simulink model "RebeccaGroup (1)"  (R2020b)
settings: Solver=VariableStepAuto  StartTime=0.0  StopTime=100  RelTol=1e-3
undefined symbols (not defined in the file): LQR
libraries: pid_lib x1
settings Model: Creator=user  LastModifiedBy=user

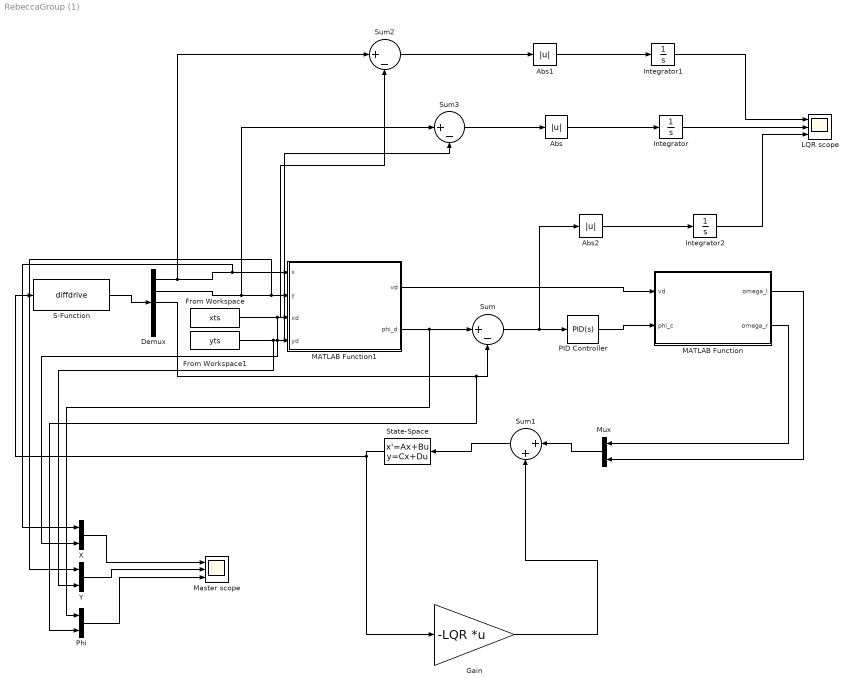
== system RebeccaGroup (1) ==
  Abs : Abs
  Abs1 : Abs
  Abs2 : Abs
  Demux : Demux  Outputs=5
  From Workspace : FromWorkspace  VariableName=xts
  From Workspace1 : FromWorkspace  VariableName=yts
  Gain : Gain  Gain=-LQR  Multiplication=Matrix(K*u)
  Integrator : Integrator
  Integrator1 : Integrator
  Integrator2 : Integrator
  LQR scope : Scope  NumInputPorts=3
  MATLAB Function : MATLAB Function  TreatAsAtomicUnit=on
  MATLAB Function1 : MATLAB Function  TreatAsAtomicUnit=on
  Master scope : Scope  NumInputPorts=3
  Mux : Mux  Inputs=2
  PID Controller : pid_lib/PID Controller  Controller=PID  Form=Parallel  TimeDomain=Continuous-time  UseExternalTs=off  SampleTime=-1  IntegratorMethod=Forward Euler  FilterMethod=Forward Euler  ControllerParametersSource=internal  P=7.98978366638355  I=11.7417923177331  D=0.804824840829485  UseFilter=on  N=170.651260101188  TunerSelectOption=Transfer Function Based (PID Tuner App)  InitialConditionSource=internal  InitialConditionForIntegrator=0  InitialConditionForFilter=0  DifferentiatorICPrevScaledInput=0  ExternalReset=none  TrackingMode=off  Kt=1  LimitOutput=off  SatLimitsSource=internal  UpperSaturationLimit=inf  LowerSaturationLimit=-inf  LinearizeAsGain=on  AntiWindupMode=none  Kb=1  POutMin=[]  POutMax=[]  IOutMin=[]  IOutMax=[]  DOutMin=[]  DOutMax=[]  NOutMin=[]  NOutMax=[]  SumOutMin=[]  SumOutMax=[]  SaturationOutMin=[]  SaturationOutMax=[]  PParamMin=[]  PParamMax=[]  IParamMin=[]  IParamMax=[]  DParamMin=[]  DParamMax=[]  NParamMin=[]  NParamMax=[]  KbParamMin=[]  KbParamMax=[]  KtParamMin=[]  KtParamMax=[]  KbOutMin=[]  KbOutMax=[]  KtOutMin=[]  KtOutMax=[]  IntegratorOutMin=[]  IntegratorOutMax=[]  FilterOutMin=[]  FilterOutMax=[]  SumI1OutMin=[]  SumI1OutMax=[]  SumI2OutMin=[]  SumI2OutMax=[]  SumI3OutMin=[]  SumI3OutMax=[]  SumI4OutMin=[]  SumI4OutMax=[]  SumDOutMin=[]  SumDOutMax=[]  DifferentiatorOutMin=[]  DifferentiatorOutMax=[]  FilterDiffOutCoefMin=[]  FilterDiffOutCoefMax=[]  ReciprocalOutMin=[]  ReciprocalOutMax=[]  SumDenOutMin=[]  SumDenOutMax=[]  SumNumOutMin=[]  SumNumOutMax=[]  DivideOutMin=[]  DivideOutMax=[]  UdiffTsProdOutMin=[]  UdiffTsProdOutMax=[]  NTsProdOutMin=[]  NTsProdOutMax=[]  UintegralTsProdOutMin=[]  UintegralTsProdOutMax=[]  UngainTsProdOutMin=[]  UngainTsProdOutMax=[]  IntegratorContinuousStateAttributes=''  IntegratorStateMustResolveToSignalObject=off  IntegratorRTWStateStorageClass=Auto  FilterContinuousStateAttributes=''  FilterStateMustResolveToSignalObject=off  FilterRTWStateStorageClass=Auto  ParallelPVariant=InternalParameters  IdealPVariant=Disabled  IVariant=InternalParameters  DVariant=InternalParameters  IntegratorVariant=Continuous  SatVariant=Disabled  AWVariant=Passthrough  PCopyVariant=Disabled  TRVariant=Disabled  FdbkBlocksVariant=Forward  IdealPFdbkVariant=Disabled  SatFdbkVariant=Disabled  DerivativeFilterVariant=ContFilter  NVariant=InternalParameters  NCopyVariant=Disabled  FilterICVariant=InternalICsFilter  IntegratorICVariant=InternalICs  ExternalResetVariant=Disabled  TRSumVariant=Passthrough  SumFdbkVariant=Disabled  SumVariant=Sum_PID  TsampFilterVariant=InternalTs  TsampNgainVariant=Passthrough  TsampIntegralVariant=Passthrough  ExternalSaturationOutDataTypeStr=Inherit: Same as second input
  Phi : Mux  Inputs=2
  S-Function : S-Function  FunctionName=diffdrive  SFunctionDeploymentMode=off  EnableBusSupport=off
  State-Space : StateSpace  A=[-10.3 0; 0 -9.4318]  B=[30 0; 0 26.5152]  C=[1 0; 0 1]  D=[0 0; 0 0]  InitialCondition=0
  Sum : Sum  Inputs=|+-
  Sum1 : Sum  Inputs=|++
  Sum2 : Sum  Inputs=|+-
  Sum3 : Sum  Inputs=|+-
  X : Mux  Inputs=2
  Y : Mux  Inputs=2
  wires:
  PID Controller/1 -> MATLAB Function/2(phi_c)
  MATLAB Function1/1(vd) -> MATLAB Function/1(vd)
  MATLAB Function1/2(phi_d) -> Phi/1, Sum/1
  Sum/1 -> Abs2/1, PID Controller/1
  S-Function/1 -> Demux/1
  Demux/1 -> Sum2/1, X/1, MATLAB Function1/1(x)
  Demux/2 -> Sum3/1, Y/1, MATLAB Function1/2(y)
  MATLAB Function/2(omega_r) -> Mux/1
  MATLAB Function/1(omega_l) -> Mux/2
  Demux/3 -> Phi/2, Sum/2
  From Workspace/1 -> Sum2/2, X/2, MATLAB Function1/3(xd)
  From Workspace1/1 -> Sum3/2, MATLAB Function1/4(yd), Y/2
  State-Space/1 -> S-Function/1, Gain/1
  Gain/1 -> Sum1/2
  Mux/1 -> Sum1/1
  Sum1/1 -> State-Space/1
  X/1 -> Master scope/1
  Y/1 -> Master scope/2
  Phi/1 -> Master scope/3
  Abs2/1 -> Integrator2/1
  Sum3/1 -> Abs/1
  Abs/1 -> Integrator/1
  Sum2/1 -> Abs1/1
  Abs1/1 -> Integrator1/1
  Integrator1/1 -> LQR scope/1
  Integrator/1 -> LQR scope/2
  Integrator2/1 -> LQR scope/3

== matlab function RebeccaGroup (1)/MATLAB Function ==
  data: omega_l output; vd input; omega_r output; phi_c input
function [omega_l, omega_r] = ActuatorMixing(vd, phi_c)

d = 4
r = 2

omega_r = (2*vd + phi_c*d)/(2*r);
omega_l = (2*vd - phi_c*d)/(2*r);

== matlab function RebeccaGroup (1)/MATLAB Function1 ==
  data: vd output; x input; phi_d output; y input; xd input; yd input
function [vd, phi_d] = TrajectoryGeneration(x, y, xd, yd)

alpha = 0.5;

phi_d = atan((yd - y)/(xd - x));
vd = alpha*(sqrt((yd - y)^2 + (xd - x)^2));

if(isnan(phi_d))
    phi_d = 0;
end
